simulink model "part2"  (R2021a)
settings: Solver=VariableStepAuto  StartTime=0.0  StopTime=100  MaxStep=1e-4  RelTol=1e-3
undefined symbols (not defined in the file): b1, b2, k1, k2, m1, m2, pulse
libraries: simulink x1
settings Model: Creator=swarn  LastModifiedBy=mansi
settings SolverCC: AlgebraicLoopSolver=TrustRegion
settings DebuggingCC: SFMachineParentedDataDiag=warning

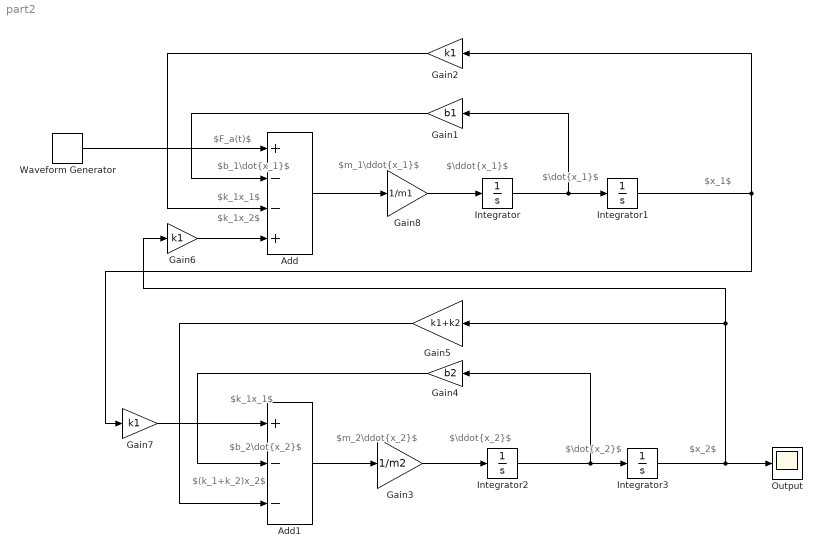
== system part2 ==
  note: $x_2$
  note: $\dot{x_2}$
  note: $\ddot{x_2}$
  note: $m_2\ddot{x_2}$
  note: $(k_1+k_2)x_2$
  note: $b_2\dot{x_2}$
  note: $k_1x_1$
  note: $k_1x_2$
  note: $k_1x_1$
  note: $b_1\dot{x_1}$
  note: $F_a(t)$
  note: $x_1$
  note: $\dot{x_1}$
  note: $\ddot{x_1}$
  note: $m_1\ddot{x_1}$
  Add : Sum  Inputs=+--+
  Add1 : Sum  Inputs=+--
  Gain1 : Gain  Gain=b1
  Gain2 : Gain  Gain=k1
  Gain3 : Gain  Gain=1/m2
  Gain4 : Gain  Gain=b2
  Gain5 : Gain  Gain=k1+k2
  Gain6 : Gain  Gain=k1
  Gain7 : Gain  Gain=k1
  Gain8 : Gain  Gain=1/m1
  Integrator{,1..3} (4 alike) : Integrator
  Output : Scope
  Waveform Generator : simulink/Sources/Waveform Generator  OutMin=[]  OutMax=[]  OutDataTypeStr=double  SelectedSignal=1  Signals=pulse(1,0,1)  BlockNames=MultiportSwitch_5d752fbb7ff64ca  SampleTime=0.1
  wires:
  Add/1 -> Gain8/1
  Integrator/1 -> Integrator1/1, Gain1/1
  Gain1/1 -> Add/2
  Integrator1/1 -> Gain2/1, Gain7/1
  Gain2/1 -> Add/3
  Add1/1 -> Gain3/1
  Integrator2/1 -> Integrator3/1, Gain4/1
  Gain4/1 -> Add1/2
  Integrator3/1 -> Output/1, Gain5/1, Gain6/1
  Gain5/1 -> Add1/3
  Gain6/1 -> Add/4
  Gain7/1 -> Add1/1
  Gain8/1 -> Integrator/1
  Gain3/1 -> Integrator2/1
  Waveform Generator/1 -> Add/1
